simulink model "Fig529"  (R2014b)
settings: Solver=ode3  StartTime=0.0  StopTime=10  FixedStep=1e-3  RelTol=1e-5
libraries: commofdm x2, commrandsrc2 x1
settings Model: Creator=Dennis Silage  LastModifiedBy=Silage
settings DataIOCC: SignalLoggingSaveFormat=ModelDataLogs
settings OptimizationCC: ExpressionDepthLimit=2147483647  InitFltsAndDblsToZero=on
settings DebuggingCC: UnderspecifiedInitializationDetection=Classic  MergeDetectMultiDrivingBlocksExec=none  SolverPrmCheckMsg=none  FcnCallInpInsideContextMsg=UseLocalSettings  StateNameClashWarn=warning
settings GRTTargetCC: CombineOutputUpdateFcns=off  GRTInterface=on

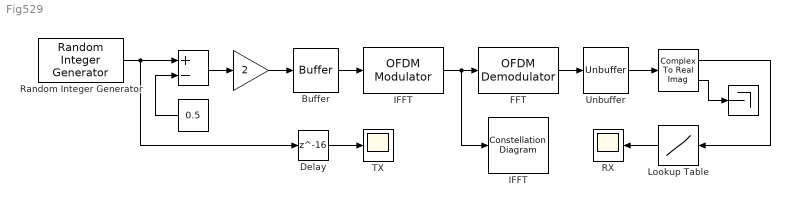
== system Fig529 ==
  "  " : ComplexToRealImag  SampleTime=1e-3
  "     " : Terminator
  "      " : Constant  Value=0.5
  "        " : Sum  Inputs=+-
  "          " : Gain  Gain=2
  "    FFT       " : commofdm/OFDM Demodulator  SimulateUsing=Interpreted execution  FFTLength=8  NumGuardBandCarriers=[0 ; 0]  RemoveDCCarrier=off  PilotOutputPort=off  PilotCarrierIndices=[12; 26; 40; 54]  CyclicPrefixLength=0  NumSymbols=1  NumReceiveAntennas=1
  "   IFFT " : commofdm/OFDM Modulator  SimulateUsing=Interpreted execution  FFTLength=8  NumGuardBandCarriers=[0 ; 0]  InsertDCNull=off  PilotInputPort=off  PilotCarrierIndices=[12; 26; 40; 54]  CyclicPrefixLength=0  Windowing=off  WindowLength=1  NumSymbols=1  NumTransmitAntennas=1
  Buffer : Buffer  N=8  TreatMby1Signals=One channel
  Delay : Delay  DelayLength=16  InitialCondition=0
  IFFT : ConstellationDiagram
  Lookup Table : Lookup_n-D  NumberOfTableDimensions=1  BreakpointsForDimension1=[-1 1]  Table=[0 1]  InternalRulePriority=Speed  RndMeth=Simplest  InputSameDT=on
  "RX " : Scope
      settings: YMin=-8  YMax=8
  Random Integer Generator : commrandsrc2/Random Integer Generator  mul=2  seed=randseed  Ts=1e-3  frameBased=off  sampPerFrame=50  orient=on  outDataType=double
  TX : Scope
      settings: YMin=-8  YMax=8  SaveName=ScopeData2
  Unbuffer : Unbuffer  SampleBasedProcessing=Same as frame based
  wires:
  "   IFFT "/1 -> IFFT/1, "    FFT       "/1
  Buffer/1 -> "   IFFT "/1
  Unbuffer/1 -> "  "/1
  "    FFT       "/1 -> Unbuffer/1
  "  "/2 -> "     "/1
  Delay/1 -> TX/1
  Random Integer Generator/1 -> Delay/1, "        "/1
  "      "/1 -> "        "/2
  "        "/1 -> "          "/1
  "          "/1 -> Buffer/1
  "  "/1 -> Lookup Table/1
  Lookup Table/1 -> "RX "/1
